simulink model "rtwdemo_profile"  (Simulink 7.6)
settings: Solver=FixedStepDiscrete  StartTime=0.0  StopTime=10.0  RelTol=1e-3
libraries: rtwdemowidgets x2, simulink x1
Description:
  | Profiling Hooks for Generated Code
settings Model: Creator=The MathWorks Inc.  ExtModeAutoUpdateStatusClock=off
settings DataIOCC: SaveOutput=off  SaveTime=off  SignalLoggingName=sigsOut
settings OptimizationCC: InlineParams=on  InlineInvariantSignals=on  StateBitsets=on  DataBitsets=on  UseTempVars=on  ZeroExternalMemoryAtStartup=off  ZeroInternalMemoryAtStartup=off  NoFixptDivByZeroProtection=on  OptimizeModelRefInitCode=on  LifeSpan=1  BufferReusableBoundary=off
settings DebuggingCC: SaveWithParameterizedLinksMsg=none  SignalResolutionControl=TryResolveAllWithWarning  SolverPrmCheckMsg=none  MultiTaskDSMMsg=warning  MultiTaskCondExecSysMsg=none  StrictBusMsg=None
settings HardwareCC: ProdBitPerLong=64  ProdEndianess=LittleEndian  ProdWordSize=64  ProdHWDeviceType=Specified  TargetHWDeviceType=32-bit Generic  ProdEqTarget=off
settings RTWCC: SystemTargetFile=ert.tlc  TLCOptions="-aProfileGenCode=1 -aProfilerTLC=\"rtwdemo_profile_hook.tlc\""  TemplateMakefile=ert_default_tmf  Description=Real-Time Workshop Embedded Coder (no auto configuration)  GenerateReport=on  RTWVerbose=off  ProcessScript=ert_make_rtw_hook  IncludeHyperlinkInReport=on  LaunchReport=on
settings CodeAppCC: ForceParamTrailComments=on  IgnoreCustomStorageClasses=off  SimulinkDataObjDesc=on  CustomSymbolStrFcn=$F$N$M  CustomSymbolStrMacro=$N$M  InsertBlockDesc=on
settings ERTTargetCC: TargetFcnLib=ansi_tfl_tmw.mat  MultiwordLength=2048  GenerateSampleERTMain=on  MatFileLogging=on  SupportComplex=off  SupportContinuousTime=on  SupportNonInlinedSFcns=on  InlinedParameterPlacement=NonHierarchical  ERTCustomFileTemplate=example_file_process.tlc  ConvertIfToSwitch=off

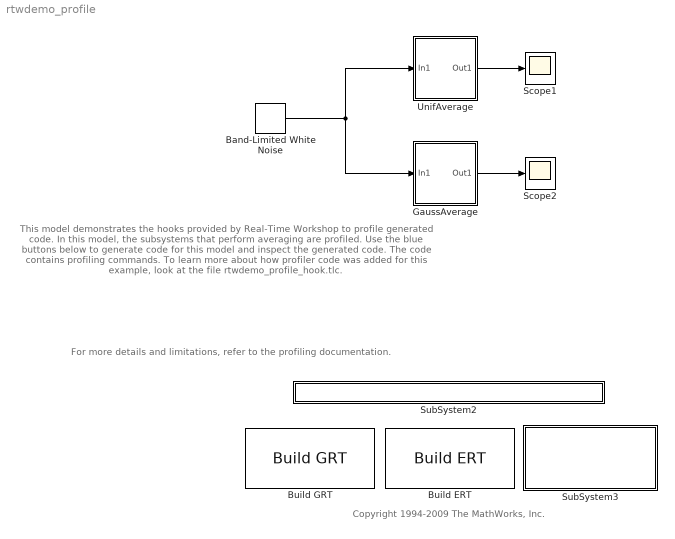
== system rtwdemo_profile ==
  note: This model demonstrates the hooks provided by Real-Time Workshop
      | to profile generated code. In this model, the subsystems that perform
      | averaging are profiled. Use the blue buttons below to generate code
      | for this model and inspect the generated code.  The code contains
      | profiling commands. To learn more about how profiler code was added
      | for this example, look at the file rtwdemo_profile_hook.tlc.
  note: Copyright 1994-2009 The MathWorks, Inc.
  note: For more details and limitations, refer to the profiling documentation.
  Band-Limited White Noise : simulink/Sources/Band-Limited White Noise  SystemSampleTime=-1  Cov=[0.1]  Ts=0.1  seed=[23341]
  Build ERT : rtwdemowidgets/Build ERT  SystemSampleTime=-1  attrib_overrides={'MatFileLogging','SupportNonFinite','IncludeMdlTerminateFcn','ERTFilePackagingFormat'}
  Build GRT : rtwdemowidgets/Build GRT  SystemSampleTime=-1  attrib_overrides={'MatFileLogging','SupportNonFinite'}
  GaussAverage : Subsystem  TreatAsAtomicUnit=on
      settings: RTWSystemCode=Function  RTWFcnNameOpts=Use subsystem name  RTWFileNameOpts=Use function name
  Scope1 : Scope
  Scope2 : Scope
  SubSystem2 : Subsystem  mask{filename=sfun_runtime3.tlc}
      mask prompts: filename "file name"
      settings: OpenFcn=edit(fullfile(matlabroot,'toolbox','rtw','rtwdemos','rtwdemo_profile_hook.tlc'))
      mask Display: disp('matlabroot\toolbox\rtw\rtwdemos\rtwdemo_profile_hook.tlc')
  SubSystem3 : Subsystem
      settings: OpenFcn=helpview(fullfile(matlabroot,'toolbox','rtw','rtwdemos','html','rtwdemo_profile_moreinfo.html'));
      mask Display: disp('View documentation\n (double-click)');
  UnifAverage : Subsystem  TreatAsAtomicUnit=on
      settings: RTWSystemCode=Function  RTWFcnNameOpts=Use subsystem name  RTWFileNameOpts=Use function name
  wires:
  Band-Limited White Noise/1 -> UnifAverage/1(In1), GaussAverage/1(In1)
  UnifAverage/1(Out1) -> Scope1/1
  GaussAverage/1(Out1) -> Scope2/1

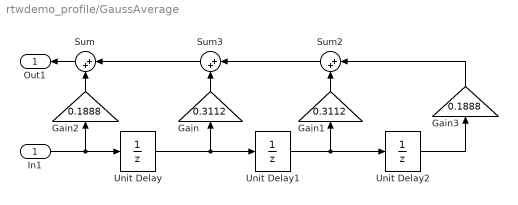
== system rtwdemo_profile/GaussAverage ==
  In1 : Inport
  Gain : Gain  Gain=0.3112  SaturateOnIntegerOverflow=on  OutDataTypeStr=Inherit: Same as input  ParamDataTypeStr=Inherit: Same as input
  Gain1 : Gain  Gain=0.3112  SaturateOnIntegerOverflow=on  OutDataTypeStr=Inherit: Same as input  ParamDataTypeStr=Inherit: Same as input
  Gain2 : Gain  Gain=0.1888  SaturateOnIntegerOverflow=on  OutDataTypeStr=Inherit: Same as input  ParamDataTypeStr=Inherit: Same as input
  Gain3 : Gain  Gain=0.1888  SaturateOnIntegerOverflow=on  OutDataTypeStr=Inherit: Same as input  ParamDataTypeStr=Inherit: Same as input
  Sum : Sum  Inputs=|++  SaturateOnIntegerOverflow=on  InputSameDT=on  OutDataTypeStr=Inherit: Same as first input
  Sum2 : Sum  Inputs=|++  SaturateOnIntegerOverflow=on  InputSameDT=on  OutDataTypeStr=Inherit: Same as first input
  Sum3 : Sum  Inputs=|++  SaturateOnIntegerOverflow=on  InputSameDT=on  OutDataTypeStr=Inherit: Same as first input
  Unit Delay : UnitDelay  SampleTime=-1
  Unit Delay1 : UnitDelay  SampleTime=-1
  Unit Delay2 : UnitDelay  SampleTime=-1
  Out1 : Outport
  wires:
  Sum/1 -> Out1/1
  Gain2/1 -> Sum/2
  In1/1 -> Unit Delay/1, Gain2/1
  Gain/1 -> Sum3/2
  Gain1/1 -> Sum2/2
  Gain3/1 -> Sum2/1
  Unit Delay2/1 -> Gain3/1
  Unit Delay1/1 -> Unit Delay2/1, Gain1/1
  Unit Delay/1 -> Gain/1, Unit Delay1/1
  Sum3/1 -> Sum/1
  Sum2/1 -> Sum3/1

== system rtwdemo_profile/SubSystem2 ==

== system rtwdemo_profile/SubSystem3 ==

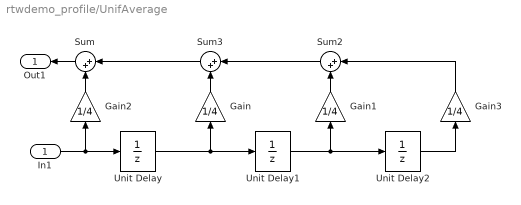
== system rtwdemo_profile/UnifAverage ==
  In1 : Inport
  Gain{,1..3} (4 alike) : Gain  Gain=1/4  SaturateOnIntegerOverflow=on  OutDataTypeStr=Inherit: Same as input  ParamDataTypeStr=Inherit: Same as input
  Sum : Sum  Inputs=|++  SaturateOnIntegerOverflow=on  InputSameDT=on  OutDataTypeStr=Inherit: Same as first input
  Sum2 : Sum  Inputs=|++  SaturateOnIntegerOverflow=on  InputSameDT=on  OutDataTypeStr=Inherit: Same as first input
  Sum3 : Sum  Inputs=|++  SaturateOnIntegerOverflow=on  InputSameDT=on  OutDataTypeStr=Inherit: Same as first input
  Unit Delay : UnitDelay  SampleTime=-1
  Unit Delay1 : UnitDelay  SampleTime=-1
  Unit Delay2 : UnitDelay  SampleTime=-1
  Out1 : Outport
  wires:
  Sum2/1 -> Sum3/1
  Sum3/1 -> Sum/1
  Unit Delay/1 -> Unit Delay1/1, Gain/1
  Unit Delay1/1 -> Unit Delay2/1, Gain1/1
  Unit Delay2/1 -> Gain3/1
  Gain3/1 -> Sum2/1
  Gain1/1 -> Sum2/2
  Gain/1 -> Sum3/2
  In1/1 -> Gain2/1, Unit Delay/1
  Gain2/1 -> Sum/2
  Sum/1 -> Out1/1
